simulink model "US_Image_Acquire_Trigger_V2"  (R2019a)
settings: Solver=FixedStepAuto  StartTime=0.0  StopTime=inf  FixedStep=Sam_time  RelTol=1e-3
values from neighbouring files (symbols this model uses):
  Epiphan_speed = round(1/Epiphan_speed,3)    [Simulink_Image_Acq_V2.m]    (also in Testing_Script.m)
  Sam_time = 0.034    [Simulink_Image_Acq.m]    (also in Simulink_Image_Acq_V2.m = round(1/Sam_time,3))
  Tot_exp_num = 8    [Simulink_Image_Acq.m]    (also in Simulink_Image_Acq_V2.m = 1)
  UDP_in = 12    [Simulink_Image_Acq.m]    (also in Simulink_Image_Acq_V2.m)
undefined symbols (not defined in the file or in its folder): Cur_exp_num, none, videoinput
libraries: powerlib_meascontrol x3, dspnetwork x2, imaqlib x1, sldrtlib x1
(part 2 of 2)

== matlab function US_Image_Acquire_Trigger_V2/MATLAB Function ==
  data: Im_new input; New_Frame output; Im_old input
function New_Frame = New_Frame(Im_new,Im_old)
tic; % Starting timer

% square_dim = [1 1 783-1 395-1];
% 
% Im_new = Im_new(square_dim(1):square_dim(1)+square_dim(3),...
%     square_dim(2):square_dim(1)+square_dim(4));
% Im_old = Im_old(square_dim(1):square_dim(1)+square_dim(3),...
%     square_dim(2):square_dim(1)+square_dim(4));

if any(sum(sum(Im_old))) && any(sum(sum(Im_new)))
    same = sum(sum(Im_new - Im_old));
    New_Frame = any(same);
else
    New_Frame = false;
end

Image = cell(1,2);
Image{1} = Im_old;
Image{2} = Im_new;

Time = toc;

% function [New_Frame,Time] = New_Frame(Im_new,Im_old)
% tic; % Starting timer
%
% square_dim = [1 1 783-1 395-1];
%
% crop_Im_new = Im_new(square_dim(1):square_dim(1)+square_dim(3),...
%     square_dim(2):square_dim(1)+square_dim(4));
% crop_Im_old = Im_old(square_dim(1):square_dim(1)+square_dim(3),...
%     square_dim(2):square_dim(1)+square_dim(4));
%
% if any(sum(sum(crop_Im_old))) && any(sum(sum(crop_Im_new)))
%     same = sum(sum(crop_Im_new - crop_Im_old));
%     New_Frame = any(same);
% else
%     New_Frame = false;
% end
%
% Time = toc;
